simulink model "sine_wave_decay"  (R2017a)
settings: Solver=VariableStepAuto  StartTime=0.0  StopTime=T  RelTol=1e-3
values from neighbouring files (symbols this model uses):
  f = 5    [MAR.m]    (also in Time_constant_new.m; corr_multi_sine.m = config(2); csd_damping_sine.m = config(2); csd_fft_testing.m = F*(0:(L/2))/L)
  Fs = 1000    [MAR.m]    (also in Time_constant_new.m; corr_multi_sine.m = config(3); csd_damping_sine.m = config(3); csd_fft_testing.m = 100)
  noise_amplitude = 1e-1    (= 0.1)    [MAR.m]    (also in Time_constant_new.m = 1e-05; csd_fft_testing.m; damping_sine.m = config(4); data_generate (PC's conflicted copy 2017-12-16).m = 1e-05)
  ramp_slope = -1    [MAR.m]    (also in Time_constant_new.m; csd_fft_testing.m; damping_sine.m = config(5); data_generate (PC's conflicted copy 2017-12-16).m)
  seed = randi([0 1000],1)    [MAR.m]    (also in TC_iteration.m; Time_constant_new.m; csd_fft_testing.m; damping_sine.m = config(8))
  tau = 0.005    [MAR.m]    (also in Time_constant_new.m; csd_fft_testing.m; damping_sine.m = config(6); data_generate (PC's conflicted copy 2017-12-16).m)
libraries: simulink x2, dspsrcs4 x1
settings Model: Creator=ljxia  LastModifiedBy=ljxia

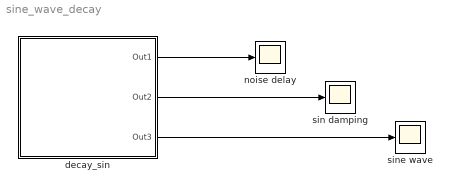
== system sine_wave_decay ==
  "decay_sin " : Subsystem
  noise delay : Scope
  sin damping : Scope
  sine wave : Scope
  wires:
  "decay_sin "/1(Out1) -> noise delay/1
  "decay_sin "/2(Out2) -> sin damping/1
  "decay_sin "/3(Out3) -> sine wave/1

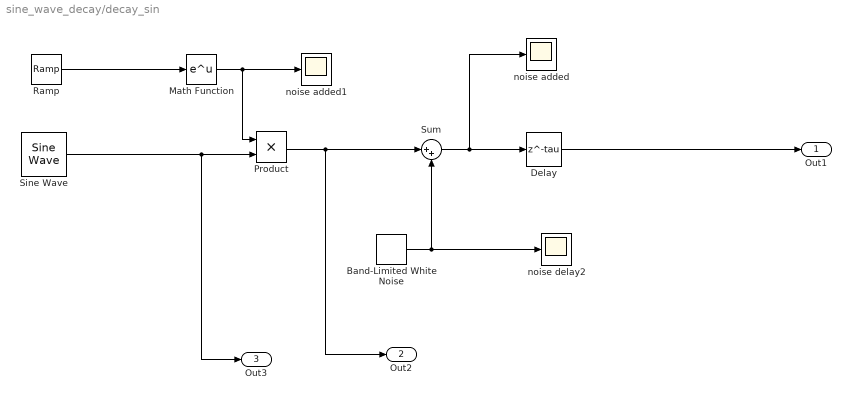
== system sine_wave_decay/decay_sin  ==
  Band-Limited White Noise : simulink/Sources/Band-Limited White Noise  Cov=[noise_amplitude]  Ts=1/Fs  seed=[seed]
  Delay : Delay  DelayLength=tau  InitialCondition=0  SampleTime=1/Fs
  Math Function : Math  SaturateOnIntegerOverflow=on
  Product : Product
  Ramp : simulink/Sources/Ramp  slope=ramp_slope  start=0  X0=0
  Sine Wave : dspsrcs4/Sine Wave  Amplitude=1  Frequency=f  Phase=0  SampleMode=Discrete  OutComplex=Real  CompMethod=Trigonometric fcn  TableSize=Speed  SampleTime=1/Fs  SamplesPerFrame=1  ResetState=Restart at time zero  OutputFrames=off  dataType=double  wordLen=16  udDataType=sfix(16)  fracBitsMode=Best precision  numFracBits=15  OutDataTypeStr=double  LastOutDataTypeStr=double
  Sum : Sum  Inputs=|++
  noise added : Scope
  noise added1 : Scope
  noise delay2 : Scope
  Out1 : Outport
  Out2 : Outport  Port=2
  Out3 : Outport  Port=3
  wires:
  Math Function/1 -> noise added1/1, Product/1
  Product/1 -> Out2/1, Sum/1
  Sum/1 -> Delay/1, noise added/1
  Sine Wave/1 -> Out3/1, Product/2
  Ramp/1 -> Math Function/1
  Band-Limited White Noise/1 -> noise delay2/1, Sum/2
  Delay/1 -> Out1/1
